simulink model "OBS6"  (Simulink 7.4)
settings: Solver=ode45  StartTime=0.0  StopTime=8  FixedStep=0.01  MinStep=0.005  RelTol=1e-3
values from neighbouring files (symbols this model uses):
  cutfreq = 2*pi    (= 6.28318530718)    [batchwamobs.m]
  K11 = 10*i11*eye(7)    [batchcontrol.m]    (also in batchwamobs.m = 15*eye(7); observer.m = 10*eye(n); observer2.m = 1000*diag([1 1 1 1 1 1]); observer3.m = 20*diag([3 4 2 1 1 1]))
  K12 = 5*i12*eye(7)    [batchcontrol.m]    (also in batchwamobs.m = 15*eye(7); observer.m = 0*eye(n); observer2.m = 0*eye(6); observer3.m = 1*eye(6))
  K21 = 5*i21*eye(7)    [batchcontrol.m]    (also in batchwamobs.m = 15*eye(7); observer.m = 0*eye(n); observer2.m = 100*eye(6); observer3.m = 1*eye(6))
  K22 = 10*i22*eye(7)    [batchcontrol.m]    (also in batchwamobs.m = 15*eye(7); observer.m = 20*eye(n); observer2.m = 100*diag([1 1 1 1 1 1]); observer3.m = 20*diag([3 4 2 1 1 1]))
  Kact = eye(7)    [batchwamobs.m]
  Kd = Kp.^0.5*2    [WAMforcecontrol.m]    (also in batchwamobs.m = 50*eye(7); paralelcontrol2R.m = eye(n)*1000)
  Kp = 25*eye(7)    [batchwamobs.m]    (also in paralelcontrol2R.m = eye(n)*2500)
  q0 = ones(n,1)*0.2    [WAMforcecontrol.m]    (also in batchwamobs.m = ones(7,1)*0.2; controltest.m = ones(7,1)*0.2; feedforward.m; paralelcontrol2R.m)
undefined symbols (not defined in the file or in its folder): model1, model2, model3, model4, model5, model6, ncalculest, observerest, p560, selectde, selectdx1e, selectdx2e, uextgenerator
libraries: roblocks x2
settings Model: Creator=acolome  LastModifiedBy=acolome

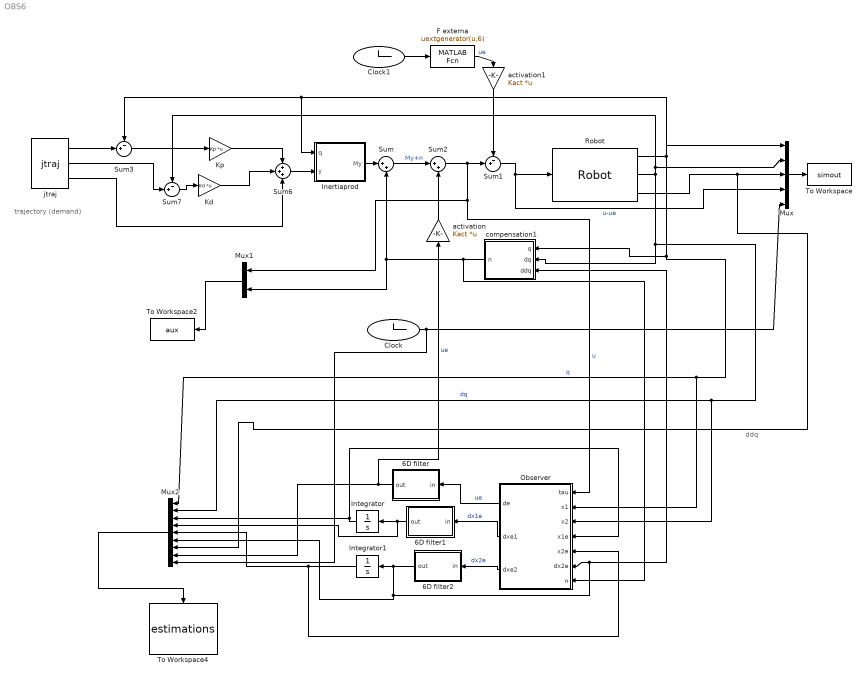
== system OBS6 ==
  note: trajectory
      | (demand)
  note: ddq
  6D filter : Subsystem  mask{K=1, tau=cutfreq}
      mask prompts: K "Gain"; tau "time constant"
  6D filter1 : Subsystem  mask{K=1, tau=cutfreq}
      mask prompts: K "Gain"; tau "time constant"
  6D filter2 : Subsystem  mask{K=1, tau=cutfreq}
      mask prompts: K "Gain"; tau "time constant"
  Clock : Clock
      settings: Decimation=100
  Clock1 : Clock
      settings: Decimation=100
  F externa : MATLABFcn  MATLABFcn=uextgenerator(u,6)  OutputDimensions=6
  Inertiaprod : Subsystem  mask{robot=p560, g=[0 0 9.81]}
      mask prompts: robot "Robot Object"; g "Gravity"
      mask init:
      | n=robot.n
      mask Display:
      | port_label('output',1,'M(q)y')
      | 
      | port_label('input', 1, 'q')
      | port_label('input', 2, 'y')
  Integrator : Integrator  InitialCondition=q0
  Integrator1 : Integrator  InitialCondition=[0 0 0 0 0 0]
  Kd : Gain  Gain=Kd  Multiplication=Matrix(K*u)  SaturateOnIntegerOverflow=on  OutDataTypeStr=Inherit: Same as input  ParamDataTypeStr=Inherit: Same as input
  Kp : Gain  Gain=Kp  Multiplication=Matrix(K*u)  SaturateOnIntegerOverflow=on  OutDataTypeStr=Inherit: Same as input  ParamDataTypeStr=Inherit: Same as input
  Mux : Mux  Inputs=5
  Mux1 : Mux  Inputs=2
  Mux2 : Mux  Inputs=9
  Observer : Subsystem  mask{robot=p560, g=[0 0 9.81], K11=K11, K12=K12, K21=K21, K22=K22}
      mask prompts: robot "Robot Object"; g "Gravity"
      mask init:
      | n=robot.n
      mask Display:
      | port_label('output',1,'de')
      | port_label('output', 2, 'dxe1')
      | port_label('output', 3, 'dxe2')
      | 
      | port_label('input', 1, 'tau')
      | port_label('input', 2, 'q')
      | port_label('input', 3, 'dq')
      | port_label('input', 4, 'x1e')
      | port_label('input', 5, 'x2e')
      | port_label('input', 6, 'dx2e')
      | port_label('input', 7, 'nest')
  Robot : roblocks/Robot  SystemSampleTime=-1  robot=p560  q0=q0
      link override Integrator1: InitialCondition=q0
  Sum : Sum  Inputs=|++  OutDataType=fixdt(1, 16)  OutScaling=2^0
  Sum1 : Sum  Inputs=-+|  OutDataType=fixdt(1, 16)  OutScaling=2^0
  Sum2 : Sum  Inputs=|++  OutDataType=fixdt(1, 16)  OutScaling=2^0
  Sum3 : Sum  Inputs=-+|  SaturateOnIntegerOverflow=on  InputSameDT=on  OutDataTypeStr=Inherit: Same as first input
  Sum6 : Sum  Inputs=+++  OutDataType=fixdt(1, 16)  OutScaling=2^0
  Sum7 : Sum  Inputs=-+|  SaturateOnIntegerOverflow=on  InputSameDT=on  OutDataTypeStr=Inherit: Same as first input
  To Workspace : ToWorkspace  VariableName=simout  SampleTime=-1  SaveFormat=Array
  To Workspace2 : ToWorkspace  VariableName=aux  SampleTime=-1  SaveFormat=Array
  To Workspace4 : ToWorkspace  VariableName=estimations  SampleTime=-1  SaveFormat=Array
  activation : Gain  Gain=Kact  Multiplication=Matrix(K*u)  SaturateOnIntegerOverflow=on  OutDataTypeStr=Inherit: Same as input  ParamDataTypeStr=Inherit: Same as input
  activation1 : Gain  Gain=Kact  Multiplication=Matrix(K*u)  SaturateOnIntegerOverflow=on  OutDataTypeStr=Inherit: Same as input  ParamDataTypeStr=Inherit: Same as input
  compensation1 : Subsystem  mask{robot=p560, g=[0 0 9.81], model1=model1, model2=model2, model3=model3, model4=model4, model5=model5, model6=model6}
      mask prompts: robot "Robot Object"; g "Gravity"; model1 "n1"; model2 "n2"; model3 "n3"; model4 "n4"; model5 "n5"; model6 "n6"
      mask init:
      | n=robot.n
      mask Display:
      | port_label('output',1,'n(q,dq)')
      | 
      | port_label('input', 1, 'q')
      | port_label('input', 2, 'dq')
      | port_label('input', 3, 'ddq')
  jtraj : roblocks/jtraj  SystemSampleTime=-1  q0=q0  qf=qf  tmax=8
      link override MATLAB Fcn: MATLABFcn=squeeze(interp1(t,q,u))
      link override MATLAB Fcn1: MATLABFcn=squeeze(interp1(t,qd,u))
      link override MATLAB Fcn2: MATLABFcn=squeeze(interp1(t,qdd,u))
  wires:
  Mux/1 -> To Workspace/1
  jtraj/2 -> Sum7/2
  Sum7/1 -> Kd/1
  Sum3/1 -> Kp/1
  jtraj/3 -> Sum6/3
  Kd/1 -> Sum6/2
  Kp/1 -> Sum6/1
  jtraj/1 -> Sum3/2
  Robot/1 -> compensation1/1(q), Mux2/1, Observer/2(x1), Inertiaprod/1(q), Sum3/1, Mux/1  "q"
  Robot/2 -> Sum7/1, Mux/2, compensation1/2(dq), Mux2/2, Observer/3(x2)  "dq"
  Sum6/1 -> Inertiaprod/2(y)
  Robot/3 -> Mux/3, Mux2/7
  Clock/1 -> Mux2/9, Mux/5
  Mux2/1 -> To Workspace4/1
  Integrator1/1 -> Mux2/5, Observer/5(x2e)
  Integrator/1 -> Mux2/3, Observer/4(x1e)
  compensation1/1(n) -> Sum/2, Mux1/2, Observer/7(n)
  6D filter/1(out) -> Mux2/8, activation/1  "ue"
  Observer/2(dxe1) -> 6D filter1/1(in)  "dx1e"
  6D filter1/1(out) -> Integrator/1, Mux2/4
  Observer/3(dxe2) -> 6D filter2/1(in)  "dx2e"
  6D filter2/1(out) -> Integrator1/1, Mux2/6, Observer/6(dx2e), compensation1/3(ddq)
  Sum1/1 -> Robot/1, Mux/4  "u-ue"
  Inertiaprod/1(My) -> Sum/1
  Clock1/1 -> F externa/1
  Sum/1 -> Sum2/1  "My+n"
  Sum2/1 -> Sum1/2, Observer/1(tau), Mux1/1  "u"
  F externa/1 -> activation1/1  "ue"
  activation1/1 -> Sum1/1
  activation/1 -> Sum2/2
  Mux1/1 -> To Workspace2/1
  Observer/1(de) -> 6D filter/1(in)  "ue"

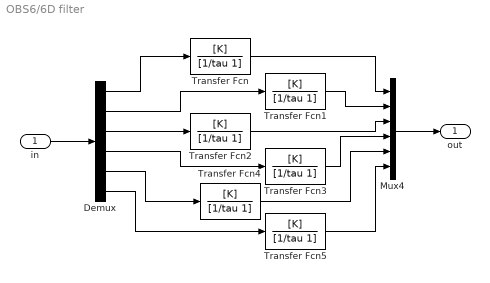
== system OBS6/6D filter ==
  in : Inport  OutDataType=fixdt(1, 16)  OutScaling=2^0
  Demux : Demux  Outputs=6
  Mux4 : Mux  Inputs=6
  Transfer Fcn{,1..5} (6 alike) : TransferFcn  Numerator=[K]  Denominator=[1/tau 1]
  out : Outport  OutDataType=fixdt(1, 16)  OutScaling=2^0
  wires:
  Demux/1 -> Transfer Fcn/1
  Demux/2 -> Transfer Fcn1/1
  Demux/3 -> Transfer Fcn2/1
  Demux/4 -> Transfer Fcn3/1
  Demux/5 -> Transfer Fcn4/1
  Demux/6 -> Transfer Fcn5/1
  Transfer Fcn/1 -> Mux4/1
  Transfer Fcn1/1 -> Mux4/2
  Transfer Fcn2/1 -> Mux4/3
  Transfer Fcn3/1 -> Mux4/4
  Transfer Fcn4/1 -> Mux4/5
  Transfer Fcn5/1 -> Mux4/6
  Mux4/1 -> out/1
  in/1 -> Demux/1

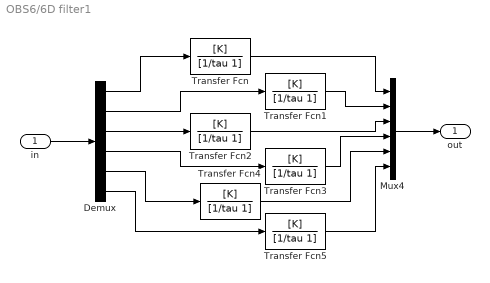
== system OBS6/6D filter1 ==
  in : Inport  OutDataType=fixdt(1, 16)  OutScaling=2^0
  Demux : Demux  Outputs=6
  Mux4 : Mux  Inputs=6
  Transfer Fcn{,1..5} (6 alike) : TransferFcn  Numerator=[K]  Denominator=[1/tau 1]
  out : Outport  OutDataType=fixdt(1, 16)  OutScaling=2^0
  wires:
  Demux/1 -> Transfer Fcn/1
  Demux/2 -> Transfer Fcn1/1
  Demux/3 -> Transfer Fcn2/1
  Demux/4 -> Transfer Fcn3/1
  Demux/5 -> Transfer Fcn4/1
  Demux/6 -> Transfer Fcn5/1
  Transfer Fcn/1 -> Mux4/1
  Transfer Fcn1/1 -> Mux4/2
  Transfer Fcn2/1 -> Mux4/3
  Transfer Fcn3/1 -> Mux4/4
  Transfer Fcn4/1 -> Mux4/5
  Transfer Fcn5/1 -> Mux4/6
  Mux4/1 -> out/1
  in/1 -> Demux/1

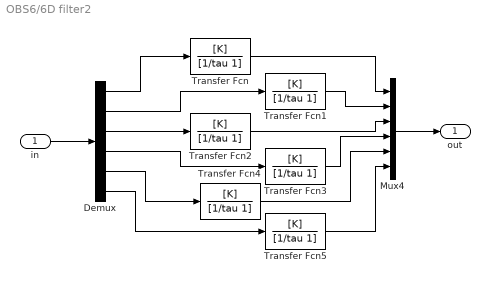
== system OBS6/6D filter2 ==
  in : Inport  OutDataType=fixdt(1, 16)  OutScaling=2^0
  Demux : Demux  Outputs=6
  Mux4 : Mux  Inputs=6
  Transfer Fcn{,1..5} (6 alike) : TransferFcn  Numerator=[K]  Denominator=[1/tau 1]
  out : Outport  OutDataType=fixdt(1, 16)  OutScaling=2^0
  wires:
  Demux/1 -> Transfer Fcn/1
  Demux/2 -> Transfer Fcn1/1
  Demux/3 -> Transfer Fcn2/1
  Demux/4 -> Transfer Fcn3/1
  Demux/5 -> Transfer Fcn4/1
  Demux/6 -> Transfer Fcn5/1
  Transfer Fcn/1 -> Mux4/1
  Transfer Fcn1/1 -> Mux4/2
  Transfer Fcn2/1 -> Mux4/3
  Transfer Fcn3/1 -> Mux4/4
  Transfer Fcn4/1 -> Mux4/5
  Transfer Fcn5/1 -> Mux4/6
  Mux4/1 -> out/1
  in/1 -> Demux/1

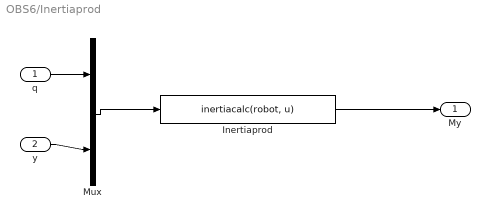
== system OBS6/Inertiaprod ==
  q : Inport  OutDataType=fixdt(1, 16)  OutScaling=2^0
  y : Inport  Port=2  OutDataType=fixdt(1, 16)  OutScaling=2^0
  Inertiaprod : MATLABFcn  MATLABFcn=inertiacalc(robot, u)  OutputDimensions=n
  Mux : Mux  Inputs=2
  My : Outport  OutDataType=fixdt(1, 16)  OutScaling=2^0
  wires:
  Mux/1 -> Inertiaprod/1
  q/1 -> Mux/1
  Inertiaprod/1 -> My/1
  y/1 -> Mux/2

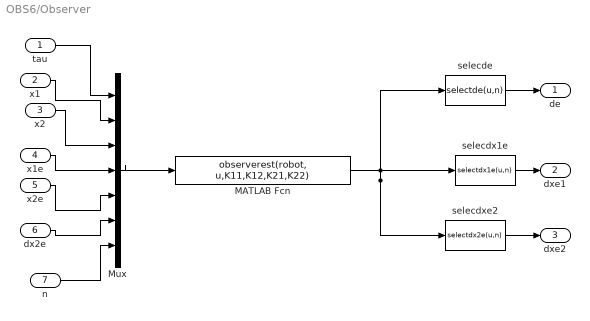
== system OBS6/Observer ==
  tau : Inport  OutDataType=fixdt(1, 16)  OutScaling=2^0
  x1 : Inport  Port=2  OutDataType=fixdt(1, 16)  OutScaling=2^0
  x2 : Inport  Port=3  OutDataType=fixdt(1, 16)  OutScaling=2^0
  x1e : Inport  Port=4  OutDataType=fixdt(1, 16)  OutScaling=2^0
  x2e : Inport  Port=5  OutDataType=fixdt(1, 16)  OutScaling=2^0
  dx2e : Inport  Port=6  OutDataType=fixdt(1, 16)  OutScaling=2^0
  n : Inport  Port=7  OutDataType=fixdt(1, 16)  OutScaling=2^0
  MATLAB Fcn : MATLABFcn  MATLABFcn=observerest(robot, u,K11,K12,K21,K22)  OutputDimensions=3*n
  Mux : Mux  Inputs=7
  selecde : MATLABFcn  MATLABFcn=selectde(u,n)
  selecdx1e : MATLABFcn  MATLABFcn=selectdx1e(u,n)
  selecdxe2 : MATLABFcn  MATLABFcn=selectdx2e(u,n)
  de : Outport  OutDataType=fixdt(1, 16)  OutScaling=2^0
  dxe1 : Outport  Port=2  OutDataType=fixdt(1, 16)  OutScaling=2^0
  dxe2 : Outport  Port=3  OutDataType=fixdt(1, 16)  OutScaling=2^0
  wires:
  Mux/1 -> MATLAB Fcn/1
  tau/1 -> Mux/1
  x1/1 -> Mux/2
  x2/1 -> Mux/3
  x1e/1 -> Mux/4
  x2e/1 -> Mux/5
  dx2e/1 -> Mux/6
  MATLAB Fcn/1 -> selecde/1, selecdx1e/1, selecdxe2/1
  selecde/1 -> de/1
  selecdx1e/1 -> dxe1/1
  selecdxe2/1 -> dxe2/1
  n/1 -> Mux/7

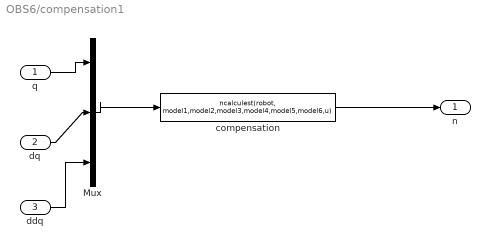
== system OBS6/compensation1 ==
  q : Inport  OutDataType=fixdt(1, 16)  OutScaling=2^0
  dq : Inport  Port=2  OutDataType=fixdt(1, 16)  OutScaling=2^0
  ddq : Inport  Port=3  OutDataType=fixdt(1, 16)  OutScaling=2^0
  Mux : Mux  Inputs=3
  compensation : MATLABFcn  MATLABFcn=ncalculest(robot, model1,model2,model3,model4,model5,model6,u)  OutputDimensions=n
  n : Outport  OutDataType=fixdt(1, 16)  OutScaling=2^0
  wires:
  Mux/1 -> compensation/1
  q/1 -> Mux/1
  compensation/1 -> n/1
  dq/1 -> Mux/2
  ddq/1 -> Mux/3
